simulink model "nonlinear"  (Simulink 9.1)
settings: Solver=VariableStepAuto  StartTime=0.0  StopTime=30  RelTol=1e-3
values from neighbouring files (symbols this model uses):
  c = 0.25    [linear_pendulum_plot.m]    (also in pendulum.m)
  g = 9.81    [linear_pendulum_plot.m]    (also in pendulum.m)
  l = 2    [linear_pendulum_plot.m]    (also in pendulum.m)
  m = 1    [linear_pendulum_plot.m]    (also in pendulum.m)
settings Model: SuppressorTable=22 serialization::archive 11 0 6 0 0 0 1 0  Creator=ee128-aaz  LastModifiedBy=ee128-aaz
settings DataIOCC: SaveFormat=Dataset
settings OptimizationCC: LifeSpan=auto
settings DebuggingCC: UnderspecifiedInitializationDetection=Simplified  MergeDetectMultiDrivingBlocksExec=error  SFUnexpectedBacktrackingDiag=error  SFNoUnconditionalDefaultTransitionDiag=error  SFExecutionAtInitializationDiag=warning
settings HardwareCC: ProdBitPerPointer=64  ProdBitPerSizeT=64  ProdBitPerPtrDiffT=64  ProdLargestAtomicFloat=Float  ProdIntDivRoundTo=Zero  ProdEndianess=LittleEndian  ProdWordSize=64  ProdHWDeviceType=Intel->x86-64 (Windows64)
settings ModelReferenceCC: PropagateSignalLabelsOutOfModel=on
settings CodeAppCC: StateflowObjectComments=off
settings GRTTargetCC: TargetLangStandard=C99 (ISO)  CombineOutputUpdateFcns=on  GRTInterface=off
settings ConfigComp: CovMetricSettings=dwe  CovHtmlReporting=off  CovSaveCumulativeToWorkspaceVar=off  CovSaveSingleToWorkspaceVar=off  CovExternalEMLEnable=on

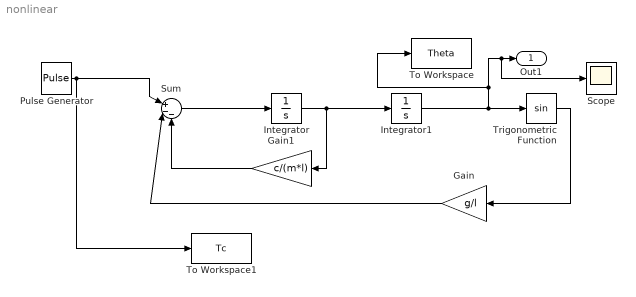
== system nonlinear ==
  Gain : Gain  Gain=g/l
  Gain1 : Gain  Gain=c/(m*l)
  Integrator : Integrator
  Integrator1 : Integrator
  Pulse Generator : DiscretePulseGenerator  PulseType=Time based  Amplitude=250  Period=100  PulseWidth=0.2
  Scope : Scope
  Sum : Sum  Inputs=|+--
  To Workspace : ToWorkspace  VariableName=Theta  SaveFormat=Timeseries  SampleTime=-1
  To Workspace1 : ToWorkspace  VariableName=Tc  SaveFormat=Timeseries  SampleTime=-1
  Trigonometric Function : Trigonometry
  Out1 : Outport
  wires:
  Sum/1 -> Integrator/1
  Integrator/1 -> Gain1/1, Integrator1/1
  Integrator1/1 -> Trigonometric Function/1, Scope/1, Out1/1, To Workspace/1
  Trigonometric Function/1 -> Gain/1
  Gain/1 -> Sum/2
  Gain1/1 -> Sum/3
  Pulse Generator/1 -> To Workspace1/1, Sum/1
